simulink model "EarthTestHarness"  (R2024a)
settings: configuration reference "standardSILConfiguraitonParams" (kept outside this file)
settings Model: Creator=jerem  LastModifiedBy=jerem
settings ConfigSetRef: SourceName=standardSILConfiguraitonParams  SourceLocation=Base Workspace

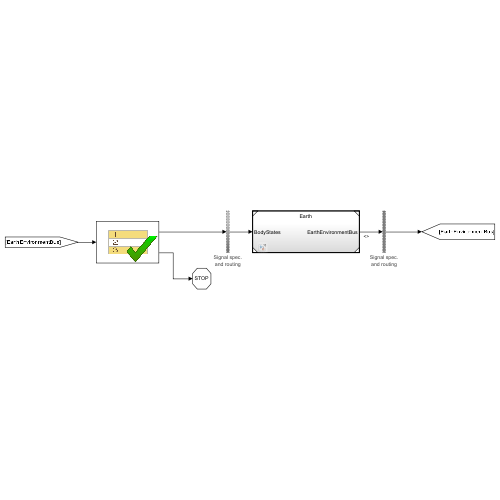
[thumbnail: Simulink's stored preview of the top-level diagram]
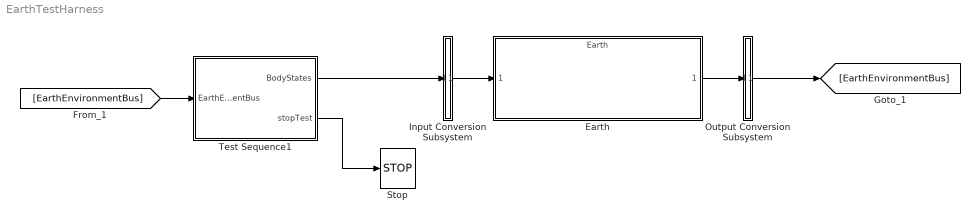
== system EarthTestHarness ==
  Earth : ModelReference  ModelNameDialog=Earth  SimulationMode=Normal  ModelReferenceVersion=1.22
  Input Conversion Subsystem : Subsystem  Tag=__SLT_ICS__  Description=|
      | Signal spec.
      | and routing
      settings: AttributesFormatString=%<Description>
  Output Conversion Subsystem : Subsystem  Tag=__SLT_OCS__  Description=|
      | Signal spec.
      | and routing
      mask init:
      | ICDictionary = get_param(bdroot, 'DataDictionary');
      | if isempty(ICDictionary)
      |    ICScope = Simulink.data.BaseWorkspace;
      | else
      |    ICScope = Simulink.data.DataDictionary(ICDictionary);
      | end
      | 
      | IC1 = Simulink.Bus.createMATLABStruct('EarthEnvironmentBus', [], [1 1], ICScope);
      settings: AttributesFormatString=%<Description>
  Stop : Stop
  Test Sequence1 : Test Sequence  TreatAsAtomicUnit=on
  wires:
  Test Sequence1/1(BodyStates) -> Input Conversion Subsystem/1(Inport_1)
  [EarthEnvironmentBus] -> Test Sequence1/1(EarthEnvironmentBus)
  Output Conversion Subsystem/1(Outport_1) -> [EarthEnvironmentBus]
  Test Sequence1/2(stopTest) -> Stop/1
  Earth/1 -> Output Conversion Subsystem/1(Inport_1)
  Input Conversion Subsystem/1(Outport_1) -> Earth/1

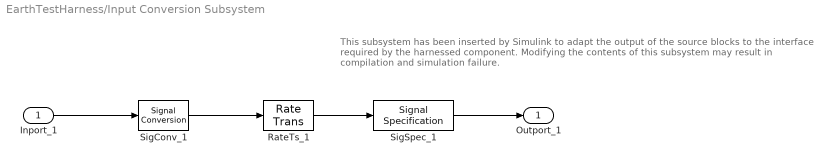
== system EarthTestHarness/Input Conversion Subsystem ==
  note: This subsystem has been inserted by Simulink to adapt the output of the source blocks to the interface required by the harnessed component.
      |  Modifying the contents of this subsystem may result in compilation and simulation failure.
  Inport_1 : Inport
  RateTs_1 : RateTransition  OutPortSampleTime=0.004
  SigConv_1 : SignalConversion  ConversionOutput=Virtual bus  OverrideOpt=off
  SigSpec_1 : SignalSpecification  OutDataTypeStr=Bus: BodyStateBus  SampleTime=0.004
  Outport_1 : Outport
  wires:
  SigSpec_1/1 -> Outport_1/1
  RateTs_1/1 -> SigSpec_1/1
  SigConv_1/1 -> RateTs_1/1
  Inport_1/1 -> SigConv_1/1

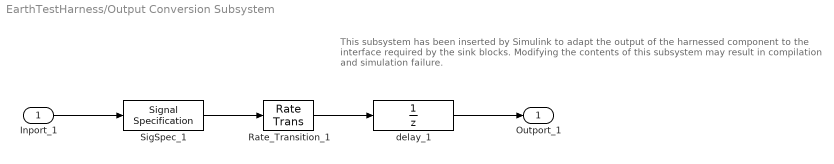
== system EarthTestHarness/Output Conversion Subsystem ==
  note: This subsystem has been inserted by Simulink to adapt the output of the harnessed component to the interface required by the sink blocks.
      |  Modifying the contents of this subsystem may result in compilation and simulation failure.
  Inport_1 : Inport
  Rate_Transition_1 : RateTransition  OutPortSampleTimeOpt=Inherit
  SigSpec_1 : SignalSpecification  OutDataTypeStr=Bus: EarthEnvironmentBus  Dimensions=[1]  SampleTime=0.004
  delay_1 : UnitDelay  InitialCondition=IC1  SampleTime=-1
  Outport_1 : Outport
  wires:
  Inport_1/1 -> SigSpec_1/1
  SigSpec_1/1 -> Rate_Transition_1/1
  Rate_Transition_1/1 -> delay_1/1
  delay_1/1 -> Outport_1/1

== stateflow chart EarthTestHarness/Test Sequence1 ==
  state Scenario_1
    state Initialize
      stopTest = false;
      BodyStates.aircraftPosInNED_m = [0;0;0];
      fieldX_nT = EarthEnvironmentBus.worldMagneticFieldInNED_nT(1);
      fieldY_nT = EarthEnvironmentBus.worldMagneticFieldInNED_nT(2);
      fieldZ_nT = EarthEnvironmentBus.worldMagneticFieldInNED_nT(3);
      gravLow_mps2 = EarthEnvironmentBus.gravityScalar_mps2;
    state changeAircraftPOSZ
      BodyStates.aircraftPosInNED_m = [100000;200000;-1000000];
    state verifyAircraftZChange
      verify(gravLow_mps2  > EarthEnvironmentBus.gravityScalar_mps2);
    state EndTest
      stopTest = true;
    (default) -> Initialize
    changeAircraftPOSZ -> verifyAircraftZChange : [
        | after(2,sec)
        | ]
    Initialize -> changeAircraftPOSZ : [
        | after(3,sec)
        | ]
    verifyAircraftZChange -> EndTest : [
        | after(2,sec)
        | ]
  (default) -> Scenario_1 : {assert(Active_Scenario_Index == 1,'The value of Scenario Parameter ''Active_Scenario_Index'' is not valid. Use the index of the scenario to specify it.')}
  data: EarthEnvironmentBus input Bus: EarthEnvironmentBus size=[1]; BodyStates output Bus: BodyStateBus size=[1]; Active_Scenario_Index parameter =1; stopTest output; gravLow_mps2 local; fieldX_nT local; fieldZ_nT local; fieldY_nT local
